simulink subsystem "CC"  (R2024a)
settings: Solver=VariableStepAuto  StartTime=0.0  StopTime=10.0  RelTol=1e-3
settings Model: Creator=nevil  LastModifiedBy=nevil

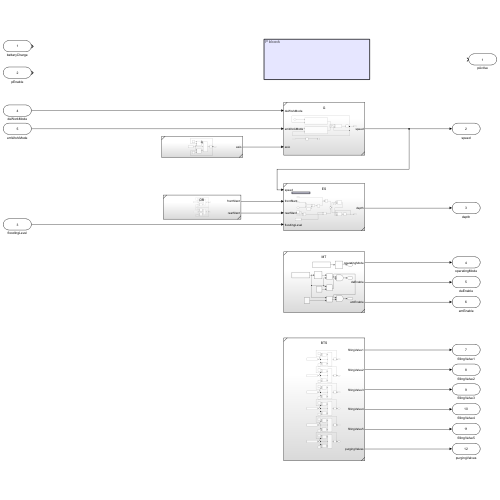
[thumbnail: Simulink's stored preview of the top-level diagram]
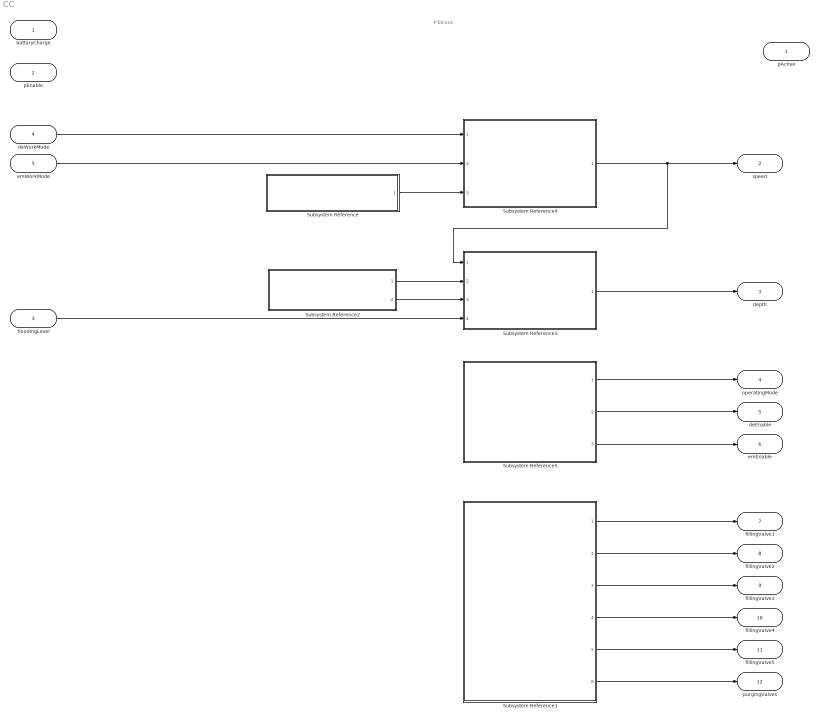
== system CC ==
  note: P blcock
  battaryCharge : Inport
  pEnable : Inport  Port=2
  floodingLevel : Inport  Port=3
  deWorkMode : Inport  Port=4
  emWorkMode : Inport  Port=5
  Subsystem Reference : Subsystem  ReferencedSubsystem=A
  Subsystem Reference1 : Subsystem  ReferencedSubsystem=BTS
  Subsystem Reference2 : Subsystem  ReferencedSubsystem=DR
  Subsystem Reference3 : Subsystem  ReferencedSubsystem=ES
  Subsystem Reference4 : Subsystem  ReferencedSubsystem=G
  Subsystem Reference5 : Subsystem  ReferencedSubsystem=MT
  pActive : Outport
  speed : Outport  Port=2
  depth : Outport  Port=3
  operatingMode : Outport  Port=4
  deEnable : Outport  Port=5
  emEnable : Outport  Port=6
  fillingValve1 : Outport  Port=7
  fillingValve2 : Outport  Port=8
  fillingValve3 : Outport  Port=9
  fillingValve4 : Outport  Port=10
  fillingValve5 : Outport  Port=11
  purgingValves : Outport  Port=12
  wires:
  Subsystem Reference4/1 -> Subsystem Reference3/1, speed/1
  Subsystem Reference2/1 -> Subsystem Reference3/2
  Subsystem Reference2/2 -> Subsystem Reference3/3
  Subsystem Reference/1 -> Subsystem Reference4/3
  floodingLevel/1 -> Subsystem Reference3/4
  deWorkMode/1 -> Subsystem Reference4/1
  emWorkMode/1 -> Subsystem Reference4/2
  Subsystem Reference3/1 -> depth/1
  Subsystem Reference5/1 -> operatingMode/1
  Subsystem Reference5/2 -> deEnable/1
  Subsystem Reference5/3 -> emEnable/1
  Subsystem Reference1/1 -> fillingValve1/1
  Subsystem Reference1/2 -> fillingValve2/1
  Subsystem Reference1/3 -> fillingValve3/1
  Subsystem Reference1/4 -> fillingValve4/1
  Subsystem Reference1/5 -> fillingValve5/1
  Subsystem Reference1/6 -> purgingValves/1
